simulink model "atrias_original"  (R2017a)
settings: Solver=ode45  StartTime=0.0  StopTime=sim_t  RelTol=1e-6  EnableMultiTasking=on
values from neighbouring files (symbols this model uses):
  N = grid_slice*1000    [createGrid.m]
  nm = fn_set_vnmc_params(sm, sample_time)    [kernel_scores_NM_mismatch.m]    (also in main_ATRIAS_cluster.m)
  nmc_BLCtrlPar = nmc.BLCtrlPar    [kernel_scores_NM_mismatch.m]    (also in main_ATRIAS_cluster.m)
  nmc_FPCtrlPar = nmc.FPCtrlPar    [kernel_scores_NM_mismatch.m]    (also in main_ATRIAS_cluster.m)
  nmc_LLCtrlPar = nmc.LLCtrlPar    [kernel_scores_NM_mismatch.m]    (also in main_ATRIAS_cluster.m)
  nmc_StCtrlPar = nmc.StCtrlPar    [kernel_scores_NM_mismatch.m]    (also in main_ATRIAS_cluster.m)
  nmc_SwCtrlPar = nmc.SwCtrlPar    [kernel_scores_NM_mismatch.m]    (also in main_ATRIAS_cluster.m)
  nmc_TrCtrlPar = nmc.TrCtrlPar    [kernel_scores_NM_mismatch.m]    (also in main_ATRIAS_cluster.m)
  nStep_switchCtrl = 10    [main_ATRIAS_cluster.m]
  nStep_thr = 1000    [createSimInitial.m]    (also in main_ATRIAS_cluster.m)
  rc_CtrlPar = [rc.k_placement, rc.T_step, rc.Cd, rc.kpt, rc.kdt, rc.desired_theta, rc.desired_z, rc.kpz, rc.kdz]    [kernel_scores_NM_mismatch.m]    (also in main_ATRIAS_cluster.m)
  sm = fn_set_MechParams(sm)    [kernel_scores_NM_mismatch.m]    (also in main_ATRIAS_cluster.m = fn_set_MechParams(sm,perturb))
  test_VNMC = 1    [createSimInitial.m]    (also in main_ATRIAS_cluster.m = 0)
undefined symbols (not defined in the file or in its folder): delta_phi_max, delta_phi_max_buffer, delta_phi_min, DiscIntNeverNeededParam, Discrete, idc, initial_dx_estimate, initial_dy_estimate, initial_dz_estimate, initial_z_estimate, kd_shin_max, kd_shin_min, kd_splay_max, kd_splay_min, kd_thigh_max, kd_thigh_min, kp_shin_max, kp_shin_min, kp_splay_max, kp_splay_min, kp_thigh_max, kp_thigh_min, mc, min_splay_angle, min_splay_buffer, phi_shin_max, phi_shin_max_buffer, phi_shin_min, phi_shin_min_buffer, phi_thigh_max, phi_thigh_max_buffer, phi_thigh_min, phi_thigh_min_buffer, rad, rc, s, sample_time, sgn, sim_d, t_friction, Time, X, Y, Z
libraries: sm_lib x202, nesl_utility x122, simulink x77, simulink_extras x24, fl_lib x16, mblibv1 x4, ctrlSharedLib x4, commnoisgen2 x1, dspswit3 x1
(part 7 of 17)

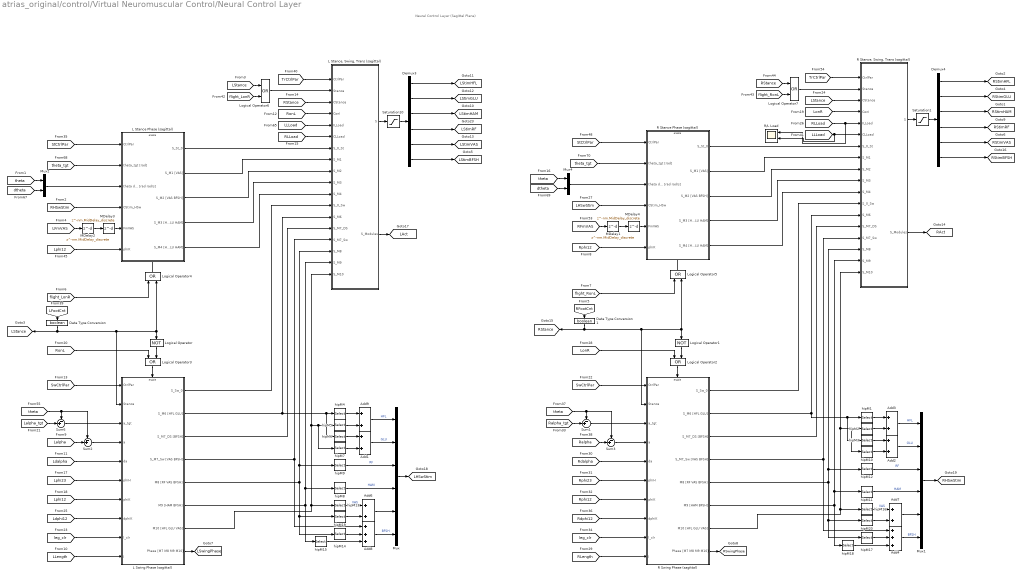
== system atrias_original/control/Virtual Neuromuscular Control/Neural Control Layer ==
  note: Neural Control Layer
      | (Sagittal Plane)
  Add{1..3,6..7,9} (6 alike) : Sum  Inputs=2
  Add4 : Sum  Inputs=3
  Add8 : Sum  Inputs=3
  Data Type Conversion : DataTypeConversion  OutDataTypeStr=boolean
  Data Type Conversion1 : DataTypeConversion  OutDataTypeStr=boolean
  Demux3 : Demux  Outputs=6
  Demux4 : Demux  Outputs=6
  L Stance Phase (sagittal) : Subsystem  TreatAsAtomicUnit=on
  "L Stance, Swing, Trans (sagittal)" : Subsystem
  L Swing Phase (sagittal) : Subsystem  TreatAsAtomicUnit=on
  Logical Operator : Logic  Operator=NOT  AllPortsSameDT=off  OutDataTypeStr=boolean
  Logical Operator1 : Logic  Operator=NOT  AllPortsSameDT=off  OutDataTypeStr=boolean
  Logical Operator{2..7} (6 alike) : Logic  Operator=OR  AllPortsSameDT=off  OutDataTypeStr=boolean
  MDelay{1..4} (4 alike) : Delay  DelayLength=nm.MidDelay_discrete  InitialCondition=0  SampleTime=sample_time
  Mux : Mux  Inputs=6
  Mux1 : Mux  Inputs=6
  Mux2 : Mux  Inputs=2
  Mux4 : Mux  Inputs=2
  R Stance Phase (sagittal) : Subsystem  TreatAsAtomicUnit=on
  "R Stance, Swing, Trans (sagittal)" : Subsystem
  R Swing Phase (sagittal) : Subsystem  TreatAsAtomicUnit=on
  R/L Load : Scope  NumInputPorts=2
  Saturation1 : Saturate  UpperLimit=1  LowerLimit=0.01  ZeroCross=off
  Saturation10 : Saturate  UpperLimit=1  LowerLimit=0.01  ZeroCross=off
  Sum{1..3,6} (4 alike) : Sum  Inputs=-+|
  hipM{1,4,8,11} (4 alike) : Selector  InputPortWidth=2  IndexOptions=Index vector (dialog)  Indices=1  OutputSizes=1
  hipM{7,10,19..20} (4 alike) : Selector  InputPortWidth=3  IndexOptions=Index vector (dialog)  Indices=2  OutputSizes=1
  hipM{2,5,9,12} (4 alike) : Selector  InputPortWidth=3  IndexOptions=Index vector (dialog)  Indices=1  OutputSizes=1
  hipM{13..14,16..17} (4 alike) : Selector  InputPortWidth=3  IndexOptions=Index vector (dialog)  Indices=3  OutputSizes=1
  hipM{3,6,15,18} (4 alike) : Selector  InputPortWidth=2  IndexOptions=Index vector (dialog)  Indices=2  OutputSizes=1
  tag scope: LAct=global, LHSwStim=global, LStance=global, LStimBFSH=global, LStimGLU=global, LStimHAM=global, LStimHFL=global, LStimRF=global, LStimVAS=global, LSwingPhase=global, RAct=global, RHSwStim=global, RStance=global, RStimBFSH=global, RStimGLU=global, RStimHAM=global, RStimHFL=global, RStimRF=global, RStimVAS=global, RSwingPhase=global
  wires:
  MDelay4/1 -> R Stance Phase (sagittal)/5(FmVAS)
  MDelay3/1 -> L Stance Phase (sagittal)/5(FmVAS)
  [RStance] -> "L Stance, Swing, Trans (sagittal)"/3(CStance)
  [RFootCnt] -> Data Type Conversion1/1
  [LFootCnt] -> Data Type Conversion/1
  [Rphi12] -> R Swing Phase (sagittal)/7(phiK)
  [Rphi23] -> R Swing Phase (sagittal)/6(phiH)
  [Rdphi12] -> R Swing Phase (sagittal)/8(dphiK)
  [Rdalpha] -> R Swing Phase (sagittal)/5(da)
  [RLength] -> R Swing Phase (sagittal)/10(l)
  Sum1/1 -> R Swing Phase (sagittal)/3(a_tgt)
  [theta] -> Sum3/1, Sum1/1
  [Ralpha_tgt] -> Sum1/2
  [leg_clr] -> R Swing Phase (sagittal)/9(l_clr)
  [Lphi12] -> L Swing Phase (sagittal)/7(phiK)
  [Lphi23] -> L Swing Phase (sagittal)/6(phiH)
  [Ldphi12] -> L Swing Phase (sagittal)/8(dphiK)
  [Ldalpha] -> L Swing Phase (sagittal)/5(da)
  [LLength] -> L Swing Phase (sagittal)/10(l)
  Add4/1 -> Mux1/6  "BFSH"
  hipM18/1 -> Add4/3
  hipM17/1 -> Add4/2
  R Swing Phase (sagittal)/3(S_M7_DS [BFSH]) -> "R Stance, Swing, Trans (sagittal)"/14(S_M7_DS)
  R Swing Phase (sagittal)/7(M10 [HFL GLU VAS]) -> "R Stance, Swing, Trans (sagittal)"/18(S_M10), hipM10/1, hipM2/1, hipM16/1
  R Swing Phase (sagittal)/5(M8 [RF VAS BFSH]) -> hipM20/1, hipM17/1, "R Stance, Swing, Trans (sagittal)"/16(S_M8), hipM12/1
  hipM15/1 -> Add8/3
  hipM14/1 -> Add8/2
  L Swing Phase (sagittal)/3(S_M7_DS [BFSH]) -> "L Stance, Swing, Trans (sagittal)"/14(S_M7_DS)
  Add8/1 -> Mux/6  "BFSH"
  "L Stance, Swing, Trans (sagittal)"/2(S_Modules) -> [LAct]
  "R Stance, Swing, Trans (sagittal)"/2(S_Modules) -> [RAct]
  R Swing Phase (sagittal)/8(Phase [M7 M8 M9 M10]) -> [RSwingPhase]
  L Swing Phase (sagittal)/8(Phase [M7 M8 M9 M10]) -> [LSwingPhase]
  hipM11/1 -> Mux1/4  "HAM"
  hipM12/1 -> Mux1/3  "RF"
  Add2/1 -> Mux1/2  "GLU"
  hipM10/1 -> Add2/2
  hipM3/1 -> Add2/1
  Add3/1 -> Mux1/1  "HFL"
  hipM2/1 -> Add3/2
  hipM1/1 -> Add3/1
  Mux1/1 -> [RHSwStim]
  R Swing Phase (sagittal)/6(M9 [HAM BFSH]) -> hipM18/1, "R Stance, Swing, Trans (sagittal)"/17(S_M9), hipM11/1
  R Swing Phase (sagittal)/2(S_M6 [HFL GLU]) -> hipM1/1, hipM3/1, "R Stance, Swing, Trans (sagittal)"/13(S_M6)
  R Swing Phase (sagittal)/1(S_Sw_0) -> "R Stance, Swing, Trans (sagittal)"/12(S_0_Sw)
  "R Stance, Swing, Trans (sagittal)"/1(S) -> Saturation1/1
  hipM8/1 -> Mux/4  "HAM"
  hipM9/1 -> Mux/3  "RF"
  Add1/1 -> Mux/2  "GLU"
  hipM7/1 -> Add1/2
  hipM6/1 -> Add1/1
  Add9/1 -> Mux/1  "HFL"
  hipM5/1 -> Add9/2
  hipM4/1 -> Add9/1
  Mux/1 -> [LHSwStim]
  L Swing Phase (sagittal)/7(M10 [HFL GLU VAS]) -> hipM7/1, hipM5/1, "L Stance, Swing, Trans (sagittal)"/18(S_M10), hipM13/1
  L Swing Phase (sagittal)/6(M9 [HAM BFSH]) -> hipM8/1, "L Stance, Swing, Trans (sagittal)"/17(S_M9), hipM15/1
  L Swing Phase (sagittal)/5(M8 [RF VAS BFSH]) -> hipM19/1, hipM14/1, hipM9/1, "L Stance, Swing, Trans (sagittal)"/16(S_M8)
  L Swing Phase (sagittal)/2(S_M6 [HFL GLU]) -> "L Stance, Swing, Trans (sagittal)"/13(S_M6), hipM4/1, hipM6/1
  L Stance Phase (sagittal)/5(S_M4 [HFL GLU HAM]) -> "L Stance, Swing, Trans (sagittal)"/11(S_M4)
  R Stance Phase (sagittal)/5(S_M4 [HFL GLU HAM]) -> "R Stance, Swing, Trans (sagittal)"/11(S_M4)
  Mux4/1 -> R Stance Phase (sagittal)/3(theta dtheta [rad rad/s])
  Mux2/1 -> L Stance Phase (sagittal)/3(theta dtheta [rad rad/s])
  [RLLoad] -> R/L Load/1, "R Stance, Swing, Trans (sagittal)"/5(ILLoad)
  R Stance Phase (sagittal)/4(S_M3 [HFL GLU HAM]) -> "R Stance, Swing, Trans (sagittal)"/10(S_M3)
  L Stance Phase (sagittal)/4(S_M3 [HFL GLU HAM]) -> "L Stance, Swing, Trans (sagittal)"/10(S_M3)
  [theta_tgt] -> R Stance Phase (sagittal)/2(theta_tgt [rad])
  [dtheta] -> Mux4/2
  [theta] -> Mux4/1
  [LLLoad] -> "L Stance, Swing, Trans (sagittal)"/5(ILLoad)
  [theta_tgt] -> L Stance Phase (sagittal)/2(theta_tgt [rad])
  [dtheta] -> Mux2/2
  [theta] -> Mux2/1
  R Stance Phase (sagittal)/3(S_M2 [VAS BFSH]) -> "R Stance, Swing, Trans (sagittal)"/9(S_M2)
  R Stance Phase (sagittal)/2(S_M1 [VAS]) -> "R Stance, Swing, Trans (sagittal)"/8(S_M1)
  L Stance Phase (sagittal)/3(S_M2 [VAS BFSH]) -> "L Stance, Swing, Trans (sagittal)"/9(S_M2)
  L Stance Phase (sagittal)/2(S_M1 [VAS]) -> "L Stance, Swing, Trans (sagittal)"/8(S_M1)
  R Stance Phase (sagittal)/1(S_St_0) -> "R Stance, Swing, Trans (sagittal)"/7(S_0_St)
  L Swing Phase (sagittal)/1(S_Sw_0) -> "L Stance, Swing, Trans (sagittal)"/12(S_0_Sw)
  L Stance Phase (sagittal)/1(S_St_0) -> "L Stance, Swing, Trans (sagittal)"/7(S_0_St)
  Sum6/1 -> L Swing Phase (sagittal)/3(a_tgt)
  [LStance] -> "R Stance, Swing, Trans (sagittal)"/3(CStance)
  Logical Operator7/1 -> "R Stance, Swing, Trans (sagittal)"/2(Stance)
  [theta] -> Sum2/1, Sum6/1
  [Lalpha_tgt] -> Sum6/2
  Demux4/6 -> [RStimBFSH]
  Demux4/5 -> [RStimVAS]
  Demux4/4 -> [RStimRF]
  Demux4/3 -> [RStimHAM]
  Demux4/2 -> [RStimGLU]
  Demux4/1 -> [RStimHFL]
  Demux3/6 -> [LStimBFSH]
  Demux3/5 -> [LStimVAS]
  Demux3/4 -> [LStimRF]
  Demux3/3 -> [LStimHAM]
  Demux3/2 -> [LStimGLU]
  Demux3/1 -> [LStimHFL]
  [RLLoad] -> "L Stance, Swing, Trans (sagittal)"/6(CLLoad)
  [LonR] -> "R Stance, Swing, Trans (sagittal)"/4(ConI)
  Saturation1/1 -> Demux4/1
  [LLLoad] -> R/L Load/2, "R Stance, Swing, Trans (sagittal)"/6(CLLoad)
  [TrCtrlPar] -> "R Stance, Swing, Trans (sagittal)"/1(CtrlPar)
  Logical Operator2/1 -> R Swing Phase (sagittal)/Enable
  Data Type Conversion1/1 -> [RStance], R Swing Phase (sagittal)/2(Stance), Logical Operator5/2, Logical Operator1/1
  [SwCtrlPar] -> R Swing Phase (sagittal)/1(CtrlPar)
  MDelay1/1 -> MDelay4/1
  [RFmVAS] -> MDelay1/1
  [LHSwStim] -> R Stance Phase (sagittal)/4(CStim_HSw)
  [StCtrlPar] -> R Stance Phase (sagittal)/1(CtrlPar)
  [RonL] -> "L Stance, Swing, Trans (sagittal)"/4(ConI)
  "L Stance, Swing, Trans (sagittal)"/1(S) -> Saturation10/1
  Saturation10/1 -> Demux3/1
  [TrCtrlPar] -> "L Stance, Swing, Trans (sagittal)"/1(CtrlPar)
  [leg_clr] -> L Swing Phase (sagittal)/9(l_clr)
  Logical Operator3/1 -> L Swing Phase (sagittal)/Enable
  Data Type Conversion/1 -> [LStance], L Swing Phase (sagittal)/2(Stance), Logical Operator/1, Logical Operator4/2
  [SwCtrlPar] -> L Swing Phase (sagittal)/1(CtrlPar)
  MDelay2/1 -> MDelay3/1
  [LFmVAS] -> MDelay2/1
  [RHSwStim] -> L Stance Phase (sagittal)/4(CStim_HSw)
  [StCtrlPar] -> L Stance Phase (sagittal)/1(CtrlPar)
  Add6/1 -> Mux/5
  hipM13/1 -> Add6/1  "VAS"
  hipM19/1 -> Add6/2
  L Swing Phase (sagittal)/4(S_M7_Sw [VAS BFSH]) -> "L Stance, Swing, Trans (sagittal)"/15(S_M7_Sw), Add8/1
  hipM20/1 -> Add7/2
  hipM16/1 -> Add7/1  "VAS"
  Add7/1 -> Mux1/5
  R Swing Phase (sagittal)/4(S_M7_Sw [VAS BFSH]) -> Add4/1, "R Stance, Swing, Trans (sagittal)"/15(S_M7_Sw)
  [Lalpha] -> Sum2/2
  Sum2/1 -> L Swing Phase (sagittal)/4(a)
  [Ralpha] -> Sum3/2
  Sum3/1 -> R Swing Phase (sagittal)/4(a)
  Logical Operator/1 -> Logical Operator3/2
  [RonL] -> Logical Operator3/1
  Logical Operator1/1 -> Logical Operator2/2
  [LonR] -> Logical Operator2/1
  Logical Operator5/1 -> R Stance Phase (sagittal)/Enable
  Logical Operator4/1 -> L Stance Phase (sagittal)/Enable
  [flight_LonR] -> Logical Operator4/1
  [flight_RonL] -> Logical Operator5/1
  [LStance] -> Logical Operator6/1
  Logical Operator6/1 -> "L Stance, Swing, Trans (sagittal)"/2(Stance)
  [flight_LonR] -> Logical Operator6/2
  [flight_RonL] -> Logical Operator7/2
  [RStance] -> Logical Operator7/1
  [Lphi12] -> L Stance Phase (sagittal)/6(phiK)
  [Rphi12] -> R Stance Phase (sagittal)/6(phiK)

== system atrias_original/control/Virtual Neuromuscular Control/Torque Distribution ==
  note: J^(-T) [tauB; tauF] = [tauH, tauK]
  note: Map Torques
  note: J^(-T) [tauB; tauF] = [tauH, tauK]
  R tauK_des [Nm] : Inport
  R tauH_des [Nm] : Inport  Port=2
  R Jacobian Constant (k) : Inport  Port=3
  L tauK_des [Nm] : Inport  Port=4
  L tauH_des [Nm] : Inport  Port=5
  L Jacobian Constant (k) : Inport  Port=6
  Demux : Demux
  Demux1 : Demux  Outputs=2
  Demux2 : Demux  Outputs=2
  L H/K torques : Scope  NumInputPorts=2
  Mux : Mux
  Mux1 : Mux  Inputs=2
  Mux2 : Mux  Inputs=2
  "R H/K torques " : Scope  NumInputPorts=2
  Switch1 : Switch  Criteria=u2 > Threshold
  Switch2 : Switch  Criteria=u2 > Threshold
  Torque Limiter (outside) {1,3..5} (4 alike) : Saturate  UpperLimit=mc.LEG_MTR_MAX_TORQUE  LowerLimit=-mc.LEG_MTR_MAX_TORQUE
      settings: AttributesFormatString=Hi: %<UpperLimit>\nLo: %<LowerLimit>
  map_tau_L : MATLAB Function  TreatAsAtomicUnit=on
  map_tau_R : MATLAB Function  TreatAsAtomicUnit=on
  mech limit avoidance1 : Subsystem  Commented=on
  R tauB [Nm] : Outport
  R tauF [Nm] : Outport  Port=2
  R J_inv_transpose [2x2] : Outport  Port=3
  L tauB [Nm] : Outport  Port=4
  L tauF [Nm] : Outport  Port=5
  L J_inv_transpose [2x2] : Outport  Port=6
  wires:
  R Jacobian Constant (k)/1 -> map_tau_R/3(k)
  map_tau_R/3(Jinv_trans) -> R J_inv_transpose [2x2]/1
  L Jacobian Constant (k)/1 -> map_tau_L/3(k)
  map_tau_L/3(Jinv_trans) -> L J_inv_transpose [2x2]/1
  map_tau_L/1(tauB) -> Mux2/1
  map_tau_L/2(tauF) -> Mux2/2
  Mux/1 -> Demux/1
  Demux/1 -> [RtauH]
  R tauH_des [Nm]/1 -> Mux/1
  R tauK_des [Nm]/1 -> Mux/2
  L tauH_des [Nm]/1 -> Mux/3
  L tauK_des [Nm]/1 -> Mux/4
  Demux/2 -> [RtauK]
  Demux/3 -> [LtauH]
  Demux/4 -> [LtauK]
  [RtauH] -> "R H/K torques "/1, map_tau_R/1(tauH_des)
  [RtauK] -> "R H/K torques "/2, map_tau_R/2(tauK_des)
  [LtauH] -> L H/K torques/1, map_tau_L/1(tauH_des)
  Switch1/1 -> Demux1/1
  [LFootCnt] -> Switch1/2
  Mux2/1 -> Torque Limiter (outside) 3/1, Torque Limiter (outside) 1/1
  Torque Limiter (outside) 3/1 -> Switch1/3
  Torque Limiter (outside) 1/1 -> Switch1/1
  Demux1/2 -> L tauF [Nm]/1
  Demux1/1 -> L tauB [Nm]/1
  map_tau_R/1(tauB) -> Mux1/1
  map_tau_R/2(tauF) -> Mux1/2
  Switch2/1 -> Demux2/1
  [RFootCnt] -> Switch2/2
  Mux1/1 -> Torque Limiter (outside) 5/1, Torque Limiter (outside) 4/1
  Torque Limiter (outside) 4/1 -> Switch2/3
  Torque Limiter (outside) 5/1 -> Switch2/1
  Demux2/2 -> R tauF [Nm]/1
  Demux2/1 -> R tauB [Nm]/1
  [LtauK] -> L H/K torques/2, map_tau_L/2(tauK_des)

== system atrias_original/ATRIAS_sim/Mechanical System Layer/Boom/Frame Data ==
  Kinematic Data : ToWorkspace  VariableName=boom_roll_out  SampleTime=sm.output_sample_time
      settings: Save2DSignal=2-D array (concatenate along first dimension)
  Mux : Mux
  PS-Simulink Converter{,1..3} (4 alike) : nesl_utility/PS-Simulink Converter  PhysicalDomain=network_engine_domain  SubClassName=ps_output  LeftPortType=input  RightPortType=output  PseudoPeriodic=off  Frequencies=[]  Unit=1  AffineConversion=off
  Transform Sensor : sm_lib/Frames and Transforms/Transform Sensor  MeasurementFrame=World  SenseAngle=off  SenseAxis=off  SenseAngle1=off  SenseAngle2=off  SenseAngle3=off  SenseQ=on  SenseR=off  SenseOmegaX=off  SenseOmegaY=off  SenseOmegaZ=off  SenseOmega1=off  SenseOmega2=off  SenseOmega3=off  SenseQDot=off  SenseRDot=off  SenseAlphaX=off  SenseAlphaY=off  SenseAlphaZ=off  SenseAlpha1=off  SenseAlpha2=off  SenseAlpha3=off  SenseQDDot=off  SenseRDDot=off  SenseX=on  SenseY=on  SenseZ=on  SenseRad=off  SenseAzim=off  SenseDist=off  SenseInc=off  SenseXDot=off  SenseYDot=off  SenseZDot=off  SenseRadDot=off  SenseAzimDot=off  SenseDistDot=off  SenseIncDot=off  SenseXDDot=off  SenseYDDot=off  SenseZDDot=off  SenseRadDDot=off  SenseAzimDDot=off  SenseDistDDot=off  SenseIncDDot=off
  World Frame : sm_lib/Frames and Transforms/World Frame
  Frame : PMIOPort  Port=1  Side=Left
  wires:
  Mux/1 -> Kinematic Data/1
  PS-Simulink Converter/1 -> Mux/1
  PS-Simulink Converter1/1 -> Mux/2
  PS-Simulink Converter2/1 -> Mux/3
  PS-Simulink Converter3/1 -> Mux/4
  connections:
  PS-Simulink Converter3/LConn1 -- Transform Sensor/RConn5
  PS-Simulink Converter2/LConn1 -- Transform Sensor/RConn4
  PS-Simulink Converter1/LConn1 -- Transform Sensor/RConn3
  PS-Simulink Converter/LConn1 -- Transform Sensor/RConn2
  Transform Sensor/RConn1 -- Frame/RConn1
  Transform Sensor/LConn1 -- World Frame/RConn1

== system atrias_original/ATRIAS_sim/Mechanical System Layer/L Ground Contact/Angle Range Map1 ==
  "[-pi, pi]" : Inport
  Constant : Constant  Value=2*pi
  Sum3 : Sum  Inputs=|++
  Switch : Switch  ZeroCross=off
  "[0,2*pi]" : Outport
  wires:
  Switch/1 -> "[0,2*pi]"/1
  Constant/1 -> Sum3/2
  Sum3/1 -> Switch/3
  "[-pi, pi]"/1 -> Switch/2, Switch/1, Sum3/1

== system atrias_original/ATRIAS_sim/Mechanical System Layer/L Ground Contact/Ground Friction Model ==
  note: Normal Ground Stiction Model
  note: Transverse Ground Friction Model
  delta normal [m] : Inport
  vnormal [m/s] : Inport  Port=2
  x [m] : Inport  Port=3
  vx [m/s] : Inport  Port=4
  z [m] : Inport  Port=5
  vz [m/s] : Inport  Port=6
  Contact! : EnablePort  StatesWhenEnabling=reset
  Data Type Conversion : DataTypeConversion  OutDataTypeStr=double
  Friction Switch : Subsystem
  Gain3 : Gain  Gain=sm.k_gy
  Gain4 : Gain  Gain=1/sm.v_gy_max
  Logical Operator : Logic  Operator=NOT  AllPortsSameDT=off  OutDataTypeStr=boolean
  Mux1 : Mux  Inputs=2
  Sum1 : Sum
  Sum2 : Sum
  normal-Axis Ground Force : Fcn  Expr="- u(1)  *  (1-u(2)) * (u(2)<1)"
  t-Axis Kinetic Friction Model : Subsystem
  t-Axis Static Friction Model : Subsystem
  FxFriction [N] : Outport  OutputWhenDisabled=reset  InitialOutput=0
      settings: AttributesFormatString=initial = '%<InitialOutput>'\nwhen\ndisabled\n'%<OutputWhenDisabled>'
  FyFriction [N] : Outport  Port=2  OutputWhenDisabled=reset  InitialOutput=0
      settings: AttributesFormatString=initial = '%<InitialOutput>'\nwhen\ndisabled\n'%<OutputWhenDisabled>'
  Fn_Ground[N] : Outport  Port=3  OutputWhenDisabled=reset  InitialOutput=0
      settings: AttributesFormatString=initial = '%<InitialOutput>'\nwhen disabled = '%<OutputWhenDisabled>'
  Stiction! : Outport  Port=4  OutputWhenDisabled=reset  InitialOutput=0
      settings: AttributesFormatString=initial = '%<InitialOutput>'\nwhen\ndisabled\n'%<OutputWhenDisabled>'
  wires:
  Data Type Conversion/1 -> Stiction!/1
  vz [m/s]/1 -> t-Axis Static Friction Model/5(vel_z [m/s]), t-Axis Kinetic Friction Model/4(vel_z [m/s])
  z [m]/1 -> t-Axis Kinetic Friction Model/3(pos_z [m]), t-Axis Static Friction Model/4(pos_z [m])
  t-Axis Kinetic Friction Model/2(posFP_z [m]) -> t-Axis Static Friction Model/7(posFP_z [m])
  Sum2/1 -> FyFriction [N]/1
  t-Axis Kinetic Friction Model/5(Fz_Slide [N]) -> Sum2/2
  t-Axis Static Friction Model/1(Fz_Stick [N]) -> Sum2/1
  Gain4/1 -> Mux1/2
  Gain3/1 -> Mux1/1
  Mux1/1 -> normal-Axis Ground Force/1
  Logical Operator/1 -> t-Axis Kinetic Friction Model/Enable
  t-Axis Kinetic Friction Model/3(Stiction!) -> Friction Switch/2(Stick!)
  t-Axis Static Friction Model/3(Sliding!) -> Friction Switch/1(Slide!)
  Friction Switch/1(Stiction) -> t-Axis Static Friction Model/Enable, Logical Operator/1, Data Type Conversion/1
  Sum1/1 -> FxFriction [N]/1
  t-Axis Static Friction Model/2(Fx_Stick [N]) -> Sum1/1
  t-Axis Kinetic Friction Model/4(Fx_Slide [N]) -> Sum1/2
  t-Axis Kinetic Friction Model/1(posFP_x [m]) -> t-Axis Static Friction Model/6(posFP_x [m])
  vx [m/s]/1 -> t-Axis Static Friction Model/3(vel_x [m/s]), t-Axis Kinetic Friction Model/2(vel_x [m/s])
  x [m]/1 -> t-Axis Static Friction Model/2(pos_x [m]), t-Axis Kinetic Friction Model/1(pos_x [m])
  vnormal [m/s]/1 -> Gain4/1
  delta normal [m]/1 -> Gain3/1
  normal-Axis Ground Force/1 -> Fn_Ground[N]/1, t-Axis Kinetic Friction Model/5(F_Normal [N]), t-Axis Static Friction Model/1(F_Normal [N])

== system atrias_original/ATRIAS_sim/Mechanical System Layer/L Ground Contact/Tranverse Component ==
  "x, y, z" : Inport
  boom yaw [rad] : Inport  Port=2
  Demux1 : Demux  Outputs=3
  Product : Product
  Product1 : Product
  Sum2 : Sum  Inputs=+|+
  Terminator1 : Terminator
  Trigonometric Function1 : Trigonometry  Operator=cos
  Trigonometric Function2 : Trigonometry
  transverse : Outport
  wires:
  Trigonometric Function2/1 -> Product1/1
  Demux1/2 -> Product1/2
  Demux1/1 -> Product/1
  Sum2/1 -> transverse/1
  Product/1 -> Sum2/1
  boom yaw [rad]/1 -> Trigonometric Function1/1, Trigonometric Function2/1
  Trigonometric Function1/1 -> Product/2
  Product1/1 -> Sum2/2
  "x, y, z"/1 -> Demux1/1
  Demux1/3 -> Terminator1/1

== system atrias_original/ATRIAS_sim/Mechanical System Layer/L Hip Shaft/Frame Data ==
  Kinematic Data : ToWorkspace  VariableName=l_hip_out  SampleTime=sm.output_sample_time
      settings: Save2DSignal=2-D array (concatenate along first dimension)
  Mux : Mux
  PS-Simulink Converter{,1..3} (4 alike) : nesl_utility/PS-Simulink Converter  PhysicalDomain=network_engine_domain  SubClassName=ps_output  LeftPortType=input  RightPortType=output  PseudoPeriodic=off  Frequencies=[]  Unit=1  AffineConversion=off
  Transform Sensor : sm_lib/Frames and Transforms/Transform Sensor  MeasurementFrame=World  SenseAngle=off  SenseAxis=off  SenseAngle1=off  SenseAngle2=off  SenseAngle3=off  SenseQ=on  SenseR=off  SenseOmegaX=off  SenseOmegaY=off  SenseOmegaZ=off  SenseOmega1=off  SenseOmega2=off  SenseOmega3=off  SenseQDot=off  SenseRDot=off  SenseAlphaX=off  SenseAlphaY=off  SenseAlphaZ=off  SenseAlpha1=off  SenseAlpha2=off  SenseAlpha3=off  SenseQDDot=off  SenseRDDot=off  SenseX=on  SenseY=on  SenseZ=on  SenseRad=off  SenseAzim=off  SenseDist=off  SenseInc=off  SenseXDot=off  SenseYDot=off  SenseZDot=off  SenseRadDot=off  SenseAzimDot=off  SenseDistDot=off  SenseIncDot=off  SenseXDDot=off  SenseYDDot=off  SenseZDDot=off  SenseRadDDot=off  SenseAzimDDot=off  SenseDistDDot=off  SenseIncDDot=off
  World Frame : sm_lib/Frames and Transforms/World Frame
  Frame : PMIOPort  Port=1  Side=Left
  wires:
  Mux/1 -> Kinematic Data/1
  PS-Simulink Converter/1 -> Mux/1
  PS-Simulink Converter1/1 -> Mux/2
  PS-Simulink Converter2/1 -> Mux/3
  PS-Simulink Converter3/1 -> Mux/4
  connections:
  PS-Simulink Converter3/LConn1 -- Transform Sensor/RConn5
  PS-Simulink Converter2/LConn1 -- Transform Sensor/RConn4
  PS-Simulink Converter1/LConn1 -- Transform Sensor/RConn3
  PS-Simulink Converter/LConn1 -- Transform Sensor/RConn2
  Transform Sensor/RConn1 -- Frame/RConn1
  Transform Sensor/LConn1 -- World Frame/RConn1

== system atrias_original/ATRIAS_sim/Mechanical System Layer/L Leg/Angle Range Map ==
  "[-pi, pi]" : Inport
  Constant : Constant  Value=2*pi
  Sum3 : Sum  Inputs=|++
  Switch : Switch  ZeroCross=off
  "[0,2*pi]" : Outport
  wires:
  Switch/1 -> "[0,2*pi]"/1
  Constant/1 -> Sum3/2
  Sum3/1 -> Switch/3
  "[-pi, pi]"/1 -> Switch/2, Switch/1, Sum3/1

== system atrias_original/ATRIAS_sim/Mechanical System Layer/L Leg/Angle Range Map1 ==
  "[-pi, pi]" : Inport
  Constant : Constant  Value=2*pi
  Sum3 : Sum  Inputs=|++
  Switch : Switch  ZeroCross=off
  "[0,2*pi]" : Outport
  wires:
  "[-pi, pi]"/1 -> Sum3/1, Switch/1, Switch/2
  Sum3/1 -> Switch/3
  Constant/1 -> Sum3/2
  Switch/1 -> "[0,2*pi]"/1

== system atrias_original/ATRIAS_sim/Mechanical System Layer/L Leg/Four Bar Link ==
  CS1 to CS2 : sm_lib/Frames and Transforms/Rigid Transform  TranslationMethod=Cartesian  TranslationStandardOffset=0  TranslationLengthUnit=m  TranslationStandardAxis=+Z  TranslationCartesianOffset=[0 -sm.l_seg 0]  TranslationROffset=0  TranslationROffsetUnits=m  TranslationZOffset=0  TranslationZOffsetUnits=m  TranslationThetaOffset=0  TranslationThetaOffsetUnits=deg  RotationMethod=None  RotationAngleUnits=deg  RotationStandardAxis=+Z  RotationAngle=0  RotationArbitraryAxis=[0 0 1]  FollAlignAxisA=+X  BaseAlignAxisA=+Y  FollAlignAxisB=+Y  BaseAlignAxisB=+Z  RotationSequenceAxes=FollowerAxes  RotationSequence=XYX  RotationSequenceAngles=[0 0 0]  RotationSequenceAnglesUnits=deg  RotationMatrix=[1 0 0; 0 1 0; 0 0 1]
  Frame Data : Subsystem
  Solid : sm_lib/Body Elements/Solid  InertiaType=Custom  Mass=sm.m_fblink  MassUnits=kg  CenterOfMass=sm.com_fblink  CenterOfMassUnits=m  MomentsOfInertia=sm.i_fblink_moments  MomentsOfInertiaUnits=kg*m^2  ProductsOfInertia=sm.i_fblink_products  ProductsOfInertiaUnits=kg*m^2  DensityBased=on  Density=1000  DensityUnits=kg/(m^3)  DoExposeReferenceFrame=on  SerializedFrames=<Frames/>  GraphicType=FromGeometry  MarkerShape=Sphere  MarkerSize=10  MarkerSizeUnits=m  GraphicVisPropType=AdvancedVisualProperties  GraphicDiffuseColor=sm.fblink_color_d  GraphicSpecularColor=[0.5 0.5 0.5 1.0]  GraphicAmbientColor=[sm.fblink_color_d*0.5 1.0]  GraphicEmissiveColor=[0.0 0.0 0.0 1.0]  GraphicShininess=128  GraphicOpacity=1.0  GeometryShape=FromFile  RectangleSize=[1 1]  RectangleSizeUnits=m  BrickDimensions="[0.1  1 0.1]"  BrickDimensionUnits=m  CylinderRadius=1  CylinderRadiusUnits=m  CylinderLength=1  CylinderLengthUnits=m  SphereRadius=1  SphereRadiusUnits=m  EllipsoidRadii=[1 1 1]  EllipsoidRadiiUnits=m  ExtrusionCrossSection=[1 1; -1 1; -1 -1; 1 -1]  ExtrusionCrossSectionUnits=m  ExtrusionLength=1  ExtrusionLengthUnits=m  PolygonNumSides=3  PolygonOuterRadius=1  PolygonOuterRadiusUnits=m  ExtGeomFileType=STL  ExtGeomFileName=../models/four_bar_link.stl  ExtGeomFileUnits=m  RevolutionCrossSection=[1 1; 1 -1; 2 -1; 2 1]  RevolutionCrossSectionUnits=m  RevolutionExtent=Full  RevolutionAngle=180  RevolutionAngleUnits=deg
  CS1 : PMIOPort  Port=1  Side=Left
  CS2 : PMIOPort  Port=2  Side=Right
  connections:
  CS1 to CS2/LConn1 -- Frame Data/LConn1 -- CS1/RConn1 -- Solid/RConn1
  CS2/RConn1 -- CS1 to CS2/RConn1

== system atrias_original/ATRIAS_sim/Mechanical System Layer/L Leg/Lower Leg ==
  CS1 to CS2 : sm_lib/Frames and Transforms/Rigid Transform  TranslationMethod=Cartesian  TranslationStandardOffset=0  TranslationLengthUnit=m  TranslationStandardAxis=+Z  TranslationCartesianOffset=[0 -sm.lowerleg_12 0]  TranslationROffset=0  TranslationROffsetUnits=m  TranslationZOffset=0  TranslationZOffsetUnits=m  TranslationThetaOffset=0  TranslationThetaOffsetUnits=deg  RotationMethod=None  RotationAngleUnits=deg  RotationStandardAxis=+Z  RotationAngle=0  RotationArbitraryAxis=[0 0 1]  FollAlignAxisA=+X  BaseAlignAxisA=+Y  FollAlignAxisB=+Y  BaseAlignAxisB=+Z  RotationSequenceAxes=FollowerAxes  RotationSequence=XYX  RotationSequenceAngles=[0 0 0]  RotationSequenceAnglesUnits=deg  RotationMatrix=[1 0 0; 0 1 0; 0 0 1]
  CS1 to CS3 : sm_lib/Frames and Transforms/Rigid Transform  TranslationMethod=Cartesian  TranslationStandardOffset=0  TranslationLengthUnit=m  TranslationStandardAxis=+Z  TranslationCartesianOffset=[0 -sm.l_seg 0]  TranslationROffset=0  TranslationROffsetUnits=m  TranslationZOffset=0  TranslationZOffsetUnits=m  TranslationThetaOffset=0  TranslationThetaOffsetUnits=deg  RotationMethod=None  RotationAngleUnits=deg  RotationStandardAxis=+Z  RotationAngle=0  RotationArbitraryAxis=[0 0 1]  FollAlignAxisA=+X  BaseAlignAxisA=+Y  FollAlignAxisB=+Y  BaseAlignAxisB=+Z  RotationSequenceAxes=FollowerAxes  RotationSequence=XYX  RotationSequenceAngles=[0 0 0]  RotationSequenceAnglesUnits=deg  RotationMatrix=[1 0 0; 0 1 0; 0 0 1]
  Frame Data : Subsystem
  Solid : sm_lib/Body Elements/Solid  InertiaType=Custom  Mass=sm.m_lowerleg  MassUnits=kg  CenterOfMass=sm.com_lowerleg  CenterOfMassUnits=m  MomentsOfInertia=sm.i_lowerleg_moments  MomentsOfInertiaUnits=kg*m^2  ProductsOfInertia=sm.i_lowerleg_products  ProductsOfInertiaUnits=kg*m^2  DensityBased=on  Density=1000  DensityUnits=kg/(m^3)  DoExposeReferenceFrame=on  SerializedFrames=<Frames/>  GraphicType=FromGeometry  MarkerShape=Sphere  MarkerSize=10  MarkerSizeUnits=m  GraphicVisPropType=AdvancedVisualProperties  GraphicDiffuseColor=sm.lowerleg_color_d  GraphicSpecularColor=[0.5 0.5 0.5 1.0]  GraphicAmbientColor=[sm.lowerleg_color_d*0.5 1.0]  GraphicEmissiveColor=[0.0 0.0 0.0 1.0]  GraphicShininess=128  GraphicOpacity=1.0  GeometryShape=FromFile  RectangleSize=[1 1]  RectangleSizeUnits=m  BrickDimensions=[0.1 1 0.1]  BrickDimensionUnits=m  CylinderRadius=1  CylinderRadiusUnits=m  CylinderLength=1  CylinderLengthUnits=m  SphereRadius=1  SphereRadiusUnits=m  EllipsoidRadii=[1 1 1]  EllipsoidRadiiUnits=m  ExtrusionCrossSection=[1 1; -1 1; -1 -1; 1 -1]  ExtrusionCrossSectionUnits=m  ExtrusionLength=1  ExtrusionLengthUnits=m  PolygonNumSides=3  PolygonOuterRadius=1  PolygonOuterRadiusUnits=m  ExtGeomFileType=STL  ExtGeomFileName=../models/lower_leg.stl  ExtGeomFileUnits=m  RevolutionCrossSection=[1 1; 1 -1; 2 -1; 2 1]  RevolutionCrossSectionUnits=m  RevolutionExtent=Full  RevolutionAngle=180  RevolutionAngleUnits=deg
  CS1 : PMIOPort  Port=1  Side=Left
  CS2 : PMIOPort  Port=2  Side=Right
  CS3 : PMIOPort  Port=3  Side=Right
  connections:
  CS2/RConn1 -- CS1 to CS2/RConn1
  CS1/RConn1 -- Frame Data/LConn1 -- Solid/RConn1 -- CS1 to CS2/LConn1 -- CS1 to CS3/LConn1
  CS3/RConn1 -- CS1 to CS3/RConn1

== system atrias_original/ATRIAS_sim/Mechanical System Layer/L Leg/Mechanical Limits ==
  note: Mechanical Limits Model
  note: Thigh-Shin Collision
  note: Thigh-Shin Flexion Collision
  dphi_shin : Inport
  phi_shin : Inport  Port=2
  dphi_thigh : Inport  Port=3
  phi_thigh : Inport  Port=4
  Compare To Constant5 : simulink/Logic and Bit Operations/Compare To Constant  relop=<=  const=sm.phi_max_collision  OutDataTypeStr=boolean  ZeroCross=off
  Compare To Zero{,1..5} (6 alike) : simulink/Logic and Bit Operations/Compare To Zero  relop=<=  OutDataTypeStr=boolean  ZeroCross=off
  Constant : Constant  Value=sm.delta_phi_min
  Constant1 : Constant  Value=sm.phi_shin_max
  Constant2 : Constant  Value=sm.phi_thigh_min
  Constant3 : Constant  Value=sm.delta_phi_max
  Constant4 : Constant  Value=sm.phi_shin_min
  Constant5 : Constant  Value=sm.phi_thigh_max
  Enabled Subsystem : Subsystem  TreatAsAtomicUnit=on
  Gain : Gain  Gain=-1
  Gain1 : Gain  Gain=-1
  Gain2 : Gain  Gain=-1
  Logical Operator : Logic  Operator=OR  Inputs=1  AllPortsSameDT=off  OutDataTypeStr=boolean
  Mux : Mux  Inputs=6
  Shin Max Collision Model : Subsystem
  Shin Min Collision Model : Subsystem
  Stop Simulation6 : Stop
  Sum{1..3,5,7} (5 alike) : Sum  Inputs=-+|
  Sum10 : Sum  Inputs=+-|
  Sum11 : Sum  Inputs=-|+
  Sum4 : Sum  Inputs=+-|
  Sum6 : Sum  Inputs=+|-
  Sum8 : Sum  Inputs=+-|
  Sum9 : Sum  Inputs=-|+
  Thigh Max Collision Model : Subsystem
  Thigh Min Collision Model : Subsystem
  Thigh-Shin Collision Model : Subsystem
  Thigh-Shin Collision Model1 : Subsystem
  tau_shin_col : Outport
  tau_thigh_shin_col : Outport  Port=2
  tau_thigh_col : Outport  Port=3
  wires:
  Compare To Zero/1 -> Thigh-Shin Collision Model/Enable
  Sum1/1 -> Sum8/2, Sum3/2
  phi_shin/1 -> Sum1/2, Sum7/2, Sum4/2
  Sum2/1 -> Gain2/1, Thigh-Shin Collision Model/2(vphi [rad/s])
  Constant/1 -> Sum3/1
  Sum3/1 -> [col_r_leg_extension], Compare To Zero/1, Thigh-Shin Collision Model/1(delta_phi [rad])
  Compare To Zero1/1 -> Shin Max Collision Model/Enable
  Constant1/1 -> Sum4/1
  phi_thigh/1 -> Sum10/2, Sum5/2, Sum1/1
  dphi_thigh/1 -> Thigh Min Collision Model/2(vphi [rad/s]), Gain1/1, Sum2/1
  Constant2/1 -> Sum5/1
  Sum5/1 -> [col_thigh_min], Compare To Zero2/1, Thigh Min Collision Model/1(phi [rad])
  Gain/1 -> Shin Max Collision Model/2(vphi [rad/s])
  Compare To Zero2/1 -> Thigh Min Collision Model/Enable
  Compare To Zero3/1 -> Thigh-Shin Collision Model1/Enable
  Constant3/1 -> Sum8/1
  Sum8/1 -> [col_r_leg_flexion], Compare To Zero3/1, Thigh-Shin Collision Model1/1(delta_phi [rad])
  Thigh-Shin Collision Model/1(tau_interaction[Nm]) -> Sum6/1
  Thigh-Shin Collision Model1/1(tau_interaction[Nm]) -> Sum6/2
  Gain2/1 -> Thigh-Shin Collision Model1/2(vphi [rad/s])
  Compare To Zero4/1 -> Shin Min Collision Model/Enable
  Constant4/1 -> Sum7/1
  Sum7/1 -> [col_shin_min], Compare To Zero4/1, Shin Min Collision Model/1(phi [rad])
  dphi_shin/1 -> Sum2/2, Gain/1, Shin Min Collision Model/2(vphi [rad/s])
  Sum9/1 -> tau_shin_col/1
  Shin Max Collision Model/1(tau_interaction[Nm]) -> Sum9/1
  Shin Min Collision Model/1(tau_interaction[Nm]) -> Sum9/2
  Sum6/1 -> tau_thigh_shin_col/1
  Constant5/1 -> Sum10/1
  Compare To Zero5/1 -> Thigh Max Collision Model/Enable
  Sum11/1 -> tau_thigh_col/1
  Thigh Min Collision Model/1(tau_interaction[Nm]) -> Sum11/2
  Gain1/1 -> Thigh Max Collision Model/2(vphi [rad/s])
  Thigh Max Collision Model/1(tau_interaction[Nm]) -> Sum11/1
  [col_thigh_max] -> Mux/1
  [col_thigh_min] -> Mux/2
  [col_shin_max] -> Mux/3
  [col_shin_min] -> Mux/4
  [col_leg_extension] -> Mux/5
  [col_r_leg_flexion] -> Mux/6
  Mux/1 -> Compare To Constant5/1
  Logical Operator/1 -> Stop Simulation6/1, Enabled Subsystem/Enable
  Sum10/1 -> Thigh Max Collision Model/1(phi [rad]), Compare To Zero5/1, [col_thigh_max]
  Sum4/1 -> [col_shin_max], Compare To Zero1/1, Shin Max Collision Model/1(phi [rad])
  Compare To Constant5/1 -> Enabled Subsystem/1(Col_Flags), Logical Operator/1

== system atrias_original/ATRIAS_sim/Mechanical System Layer/L Leg/Shin ==
  CS1 to CS2 : sm_lib/Frames and Transforms/Rigid Transform  TranslationMethod=Cartesian  TranslationStandardOffset=0  TranslationLengthUnit=m  TranslationStandardAxis=+Z  TranslationCartesianOffset=[0 -sm.shin_12 0]  TranslationROffset=0  TranslationROffsetUnits=m  TranslationZOffset=0  TranslationZOffsetUnits=m  TranslationThetaOffset=0  TranslationThetaOffsetUnits=deg  RotationMethod=None  RotationAngleUnits=deg  RotationStandardAxis=+Z  RotationAngle=0  RotationArbitraryAxis=[0 0 1]  FollAlignAxisA=+X  BaseAlignAxisA=+Y  FollAlignAxisB=+Y  BaseAlignAxisB=+Z  RotationSequenceAxes=FollowerAxes  RotationSequence=XYX  RotationSequenceAngles=[0 0 0]  RotationSequenceAnglesUnits=deg  RotationMatrix=[1 0 0; 0 1 0; 0 0 1]
  Frame Data : Subsystem
  Solid : sm_lib/Body Elements/Solid  InertiaType=Custom  Mass=sm.m_shin  MassUnits=kg  CenterOfMass=sm.com_shin  CenterOfMassUnits=m  MomentsOfInertia=sm.i_shin_moments  MomentsOfInertiaUnits=kg*m^2  ProductsOfInertia=sm.i_shin_products  ProductsOfInertiaUnits=kg*m^2  DensityBased=on  Density=1000  DensityUnits=kg/(m^3)  DoExposeReferenceFrame=on  SerializedFrames=<Frames/>  GraphicType=FromGeometry  MarkerShape=Sphere  MarkerSize=10  MarkerSizeUnits=m  GraphicVisPropType=AdvancedVisualProperties  GraphicDiffuseColor=sm.shin_color_d  GraphicSpecularColor=[0.5 0.5 0.5 1.0]  GraphicAmbientColor=[sm.shin_color_d*0.5 1.0]  GraphicEmissiveColor=[0.0 0.0 0.0 1.0]  GraphicShininess=128  GraphicOpacity=1.0  GeometryShape=FromFile  RectangleSize=[1 1]  RectangleSizeUnits=m  BrickDimensions=[1 1 1]  BrickDimensionUnits=m  CylinderRadius=1  CylinderRadiusUnits=m  CylinderLength=1  CylinderLengthUnits=m  SphereRadius=1  SphereRadiusUnits=m  EllipsoidRadii=[1 1 1]  EllipsoidRadiiUnits=m  ExtrusionCrossSection=[1 1; -1 1; -1 -1; 1 -1]  ExtrusionCrossSectionUnits=m  ExtrusionLength=1  ExtrusionLengthUnits=m  PolygonNumSides=3  PolygonOuterRadius=1  PolygonOuterRadiusUnits=m  ExtGeomFileType=STL  ExtGeomFileName=../models/shin.stl  ExtGeomFileUnits=m  RevolutionCrossSection=[1 1; 1 -1; 2 -1; 2 1]  RevolutionCrossSectionUnits=m  RevolutionExtent=Full  RevolutionAngle=180  RevolutionAngleUnits=deg
  CS1 : PMIOPort  Port=1  Side=Left
  CS2 : PMIOPort  Port=2  Side=Right
  connections:
  CS2/RConn1 -- CS1 to CS2/RConn1
  Solid/RConn1 -- Frame Data/LConn1 -- CS1/RConn1 -- CS1 to CS2/LConn1

== system atrias_original/ATRIAS_sim/Mechanical System Layer/L Leg/Shin SEA ==
  note: Shin SEA Mechanics
  Shin Gear Torque [Nm] : Inport
  Shin Joint [rad rad/s] : Inport  Port=2
  Continuous Angle : mblibv1/Utilities/Continuous Angle  rad=rad  rads=rad/s
      settings: SourceProductName=Simscape Multibody  SourceProductBaseCode=MS
  Demux : Demux  Outputs=2
  Gain : Gain  Gain=sm.k_leg_spring
  Gain1 : Gain  Gain=sm.b_leg_spring
  Initial Gear Angle : Constant  Value=sm.shin_initial_l-sm.initial_deflection_l
  Inverse Gear Ratio1 : Gain  Gain=1/sm.N
  Inverse Gear Ratio2 : Gain  Gain=sm.Kt_leg
  Inverse Gear Ratio3 : Gain  Gain=1/sm.Kt_leg
  Motor Direction : Gain  Gain=-1
  Motor Efficiency : Gain  Gain=sm.mu_motor
  Motor Controller : Subsystem  Commented=on
  Motor Electromagnetism : Subsystem  Commented=on
  Rotor Damping : Gain  Gain=sm.b_rotor
  Rotor and Gearing : Subsystem
  Sum : Sum  Inputs=++|
  Sum2 : Sum  Inputs=+|-
  Sum3 : Sum  Inputs=|+-
  Sum4 : Sum  Inputs=+|-
  Sum5 : Sum  Inputs=|++
  Torque Limiter (outside) 2 : Saturate  UpperLimit=sm.LEG_MTR_MAX_TORQUE  LowerLimit=-sm.LEG_MTR_MAX_TORQUE  ZeroCross=off
      settings: AttributesFormatString=Hi: %<UpperLimit>\nLo: %<LowerLimit>
  Rotor Joint Conn : PMIOPort  Port=1  Side=Left
  Shin Joint Torque [Nm] : Outport
  Shin Gear [rad] : Outport  Port=2
  wires:
  Continuous Angle/1 -> Sum/2
  Rotor and Gearing/2(Gearhead Velocity [rad/s]) -> Continuous Angle/2, Sum4/1
  Rotor and Gearing/1(Gearhead Position [rad]) -> Continuous Angle/1
  Sum5/1 -> Shin Joint Torque [Nm]/1, Rotor and Gearing/2(Spring Torque [Nm])
  Torque Limiter (outside) 2/1 -> Inverse Gear Ratio1/1
  Rotor and Gearing/3(Rotor Velocity [rad/s]) -> Rotor Damping/1
  Motor Efficiency/1 -> Rotor and Gearing/1(Rotor Torque [Nm])
  Inverse Gear Ratio1/1 -> Inverse Gear Ratio3/1
  Motor Electromagnetism/1(Current [A]) -> Motor Controller/2(Measured Current [A])
  Motor Controller/1(Voltage [V]) -> Motor Electromagnetism/1(Voltage [V])
  Inverse Gear Ratio2/1 -> Sum3/1
  Inverse Gear Ratio3/1 -> Inverse Gear Ratio2/1
  Rotor Damping/1 -> Sum3/2
  Sum3/1 -> Motor Efficiency/1
  Shin Gear Torque [Nm]/1 -> Motor Direction/1
  Sum/1 -> Shin Gear [rad]/1, Sum2/1
  Initial Gear Angle/1 -> Sum/1
  Demux/2 -> Sum4/2
  Demux/1 -> Sum2/2
  Shin Joint [rad rad/s]/1 -> Demux/1
  Sum4/1 -> Gain1/1
  Gain1/1 -> Sum5/2
  Gain/1 -> Sum5/1  "tau_load"
  Sum2/1 -> Gain/1
  Motor Direction/1 -> Torque Limiter (outside) 2/1
  connections:
  Rotor and Gearing/LConn1 -- Rotor Joint Conn/RConn1

== system atrias_original/ATRIAS_sim/Mechanical System Layer/L Leg/Thigh ==
  CS1 to CS2 : sm_lib/Frames and Transforms/Rigid Transform  TranslationMethod=Cartesian  TranslationStandardOffset=0  TranslationLengthUnit=m  TranslationStandardAxis=+Z  TranslationCartesianOffset=[0 -sm.l_seg 0]  TranslationROffset=0  TranslationROffsetUnits=m  TranslationZOffset=0  TranslationZOffsetUnits=m  TranslationThetaOffset=0  TranslationThetaOffsetUnits=deg  RotationMethod=None  RotationAngleUnits=deg  RotationStandardAxis=+Z  RotationAngle=0  RotationArbitraryAxis=[0 0 1]  FollAlignAxisA=+X  BaseAlignAxisA=+Y  FollAlignAxisB=+Y  BaseAlignAxisB=+Z  RotationSequenceAxes=FollowerAxes  RotationSequence=XYX  RotationSequenceAngles=[0 0 0]  RotationSequenceAnglesUnits=deg  RotationMatrix=[1 0 0; 0 1 0; 0 0 1]
  Frame Data : Subsystem
  Solid : sm_lib/Body Elements/Solid  InertiaType=Custom  Mass=sm.m_thigh  MassUnits=kg  CenterOfMass=sm.com_thigh  CenterOfMassUnits=m  MomentsOfInertia=sm.i_thigh_moments  MomentsOfInertiaUnits=kg*m^2  ProductsOfInertia=sm.i_thigh_products  ProductsOfInertiaUnits=kg*m^2  DensityBased=on  Density=1000  DensityUnits=kg/(m^3)  DoExposeReferenceFrame=on  SerializedFrames=<Frames/>  GraphicType=FromGeometry  MarkerShape=Sphere  MarkerSize=10  MarkerSizeUnits=m  GraphicVisPropType=AdvancedVisualProperties  GraphicDiffuseColor=sm.thigh_color_d  GraphicSpecularColor=[0.5 0.5 0.5 1.0]  GraphicAmbientColor=[sm.thigh_color_d*0.5 1.0]  GraphicEmissiveColor=[0.0 0.0 0.0 1.0]  GraphicShininess=128  GraphicOpacity=1.0  GeometryShape=FromFile  RectangleSize=[1 1]  RectangleSizeUnits=m  BrickDimensions=[1 1 1]  BrickDimensionUnits=m  CylinderRadius=1  CylinderRadiusUnits=m  CylinderLength=1  CylinderLengthUnits=m  SphereRadius=1  SphereRadiusUnits=m  EllipsoidRadii=[1 1 1]  EllipsoidRadiiUnits=m  ExtrusionCrossSection=[1 1; -1 1; -1 -1; 1 -1]  ExtrusionCrossSectionUnits=m  ExtrusionLength=1  ExtrusionLengthUnits=m  PolygonNumSides=3  PolygonOuterRadius=1  PolygonOuterRadiusUnits=m  ExtGeomFileType=STL  ExtGeomFileName=../models/thigh.stl  ExtGeomFileUnits=m  RevolutionCrossSection=[1 1; 1 -1; 2 -1; 2 1]  RevolutionCrossSectionUnits=m  RevolutionExtent=Full  RevolutionAngle=180  RevolutionAngleUnits=deg
  CS1 : PMIOPort  Port=1  Side=Left
  CS2 : PMIOPort  Port=2  Side=Right
  connections:
  CS1/RConn1 -- Frame Data/LConn1 -- Solid/RConn1 -- CS1 to CS2/LConn1
  CS2/RConn1 -- CS1 to CS2/RConn1

== system atrias_original/ATRIAS_sim/Mechanical System Layer/L Leg/Thigh SEA ==
  note: Thigh SEA Mechanics
  Thigh Gear Torque [Nm] : Inport
  Thigh Joint [rad rad/s] : Inport  Port=2
  Continuous Angle : mblibv1/Utilities/Continuous Angle  rad=rad  rads=rad/s
      settings: SourceProductName=Simscape Multibody  SourceProductBaseCode=MS
  Demux : Demux  Outputs=2
  Gain : Gain  Gain=sm.k_leg_spring
  Gain1 : Gain  Gain=sm.b_leg_spring
  Initial Gear Angle : Constant  Value=sm.thigh_initial_l+sm.initial_deflection_l
  Inverse Gear Ratio1 : Gain  Gain=1/sm.N
  Inverse Gear Ratio2 : Gain  Gain=sm.Kt_leg
  Inverse Gear Ratio3 : Gain  Gain=1/sm.Kt_leg
  Motor Direction : Gain  Gain=-1
  Motor Efficiency : Gain  Gain=sm.mu_motor
  Motor Controller : Subsystem  Commented=on
  Motor Electromagnetism : Subsystem  Commented=on
  Rotor Damping : Gain  Gain=sm.b_rotor
  Rotor and Gearing : Subsystem
  Sum : Sum  Inputs=++|
  Sum2 : Sum  Inputs=+|-
  Sum3 : Sum  Inputs=|+-
  Sum4 : Sum  Inputs=+|-
  Sum5 : Sum  Inputs=|++
  Torque Limiter (outside) 2 : Saturate  UpperLimit=sm.LEG_MTR_MAX_TORQUE  LowerLimit=-sm.LEG_MTR_MAX_TORQUE  ZeroCross=off
      settings: AttributesFormatString=Hi: %<UpperLimit>\nLo: %<LowerLimit>
  Rotor Joint Conn : PMIOPort  Port=1  Side=Left
  Thigh Joint Torque [Nm] : Outport
  Thigh Gear [rad] : Outport  Port=2
  wires:
  Torque Limiter (outside) 2/1 -> Inverse Gear Ratio1/1
  Rotor and Gearing/3(Rotor Velocity [rad/s]) -> Rotor Damping/1
  Sum5/1 -> Rotor and Gearing/2(Spring Torque [Nm]), Thigh Joint Torque [Nm]/1
  Rotor and Gearing/2(Gearhead Velocity [rad/s]) -> Continuous Angle/2, Sum4/1
  Motor Efficiency/1 -> Rotor and Gearing/1(Rotor Torque [Nm])
  Inverse Gear Ratio1/1 -> Inverse Gear Ratio3/1
  Thigh Gear Torque [Nm]/1 -> Motor Direction/1
  Motor Electromagnetism/1(Current [A]) -> Motor Controller/2(Measured Current [A])
  Motor Controller/1(Voltage [V]) -> Motor Electromagnetism/1(Voltage [V])
  Rotor and Gearing/1(Gearhead Position [rad]) -> Continuous Angle/1
  Continuous Angle/1 -> Sum/2
  Sum/1 -> Sum2/1, Thigh Gear [rad]/1
  Initial Gear Angle/1 -> Sum/1
  Inverse Gear Ratio2/1 -> Sum3/1
  Inverse Gear Ratio3/1 -> Inverse Gear Ratio2/1
  Demux/2 -> Sum4/2
  Demux/1 -> Sum2/2
  Thigh Joint [rad rad/s]/1 -> Demux/1
  Sum4/1 -> Gain1/1
  Gain1/1 -> Sum5/2
  Gain/1 -> Sum5/1  "tau_load"
  Rotor Damping/1 -> Sum3/2
  Sum3/1 -> Motor Efficiency/1
  Sum2/1 -> Gain/1
  Motor Direction/1 -> Torque Limiter (outside) 2/1
  connections:
  Rotor and Gearing/LConn1 -- Rotor Joint Conn/RConn1

== system atrias_original/ATRIAS_sim/Mechanical System Layer/Left Hip Roll Joint/Mechanical Limits  ==
  vphi : Inport
  phi : Inport  Port=2
  Compare To Constant5 : simulink/Logic and Bit Operations/Compare To Constant  relop=<=  const=sm.phi_max_collision  OutDataTypeStr=boolean  ZeroCross=off
  Compare To Zero1 : simulink/Logic and Bit Operations/Compare To Zero  relop=<=  OutDataTypeStr=boolean  ZeroCross=off
  Compare To Zero2 : simulink/Logic and Bit Operations/Compare To Zero  relop=<=  OutDataTypeStr=boolean  ZeroCross=off
  Constant1 : Constant  Value=sm.phi_roll_min
  Constant2 : Constant  Value=sm.phi_roll_max
  Enabled Subsystem : Subsystem  TreatAsAtomicUnit=on
  Gain2 : Gain  Gain=-1
  Logical Operator : Logic  Operator=OR  Inputs=1  AllPortsSameDT=off  OutDataTypeStr=boolean
  Mux : Mux  Inputs=2
  Roll Max Collision Model : Subsystem
  Roll Min Collision Model : Subsystem
  Stop Simulation6 : Stop
  Sum1 : Sum  Inputs=-+|
  Sum11 : Sum  Inputs=-|+
  Sum5 : Sum  Inputs=+-|
  tau_reaction : Outport
  wires:
  Gain2/1 -> Roll Max Collision Model/2(vphi [rad/s])
  vphi/1 -> Gain2/1, Roll Min Collision Model/2(vphi [rad/s])
  Roll Max Collision Model/1(tau_interaction[Nm]) -> Sum11/1
  Compare To Zero2/1 -> Roll Max Collision Model/Enable
  Sum5/1 -> Roll Max Collision Model/1(phi [rad]), Compare To Zero2/1, [col_hip_max]
  Constant2/1 -> Sum5/1
  Compare To Constant5/1 -> Logical Operator/1, Enabled Subsystem/1(Col_Flags)
  Constant1/1 -> Sum1/1
  Sum11/1 -> tau_reaction/1
  [col_hip_min] -> Mux/2
  Mux/1 -> Compare To Constant5/1
  [col_hip_max] -> Mux/1
  Logical Operator/1 -> Stop Simulation6/1, Enabled Subsystem/Enable
  phi/1 -> Sum5/2, Sum1/2
  Compare To Zero1/1 -> Roll Min Collision Model/Enable
  Roll Min Collision Model/1(tau_interaction[Nm]) -> Sum11/2
  Sum1/1 -> Roll Min Collision Model/1(phi [rad]), Compare To Zero1/1, [col_hip_min]

== system atrias_original/ATRIAS_sim/Mechanical System Layer/R Ground Contact/Angle Range Map1 ==
  "[-pi, pi]" : Inport
  Constant : Constant  Value=2*pi
  Sum3 : Sum  Inputs=|++
  Switch : Switch  ZeroCross=off
  "[0,2*pi]" : Outport
  wires:
  "[-pi, pi]"/1 -> Sum3/1, Switch/1, Switch/2
  Sum3/1 -> Switch/3
  Constant/1 -> Sum3/2
  Switch/1 -> "[0,2*pi]"/1

== system atrias_original/ATRIAS_sim/Mechanical System Layer/R Ground Contact/Ground Friction Model ==
  note: Transverse Ground Friction Model
  note: Normal Ground Stiction Model
  delta normal [m] : Inport
  vnormal [m/s] : Inport  Port=2
  x [m] : Inport  Port=3
  vx [m/s] : Inport  Port=4
  z [m] : Inport  Port=5
  vz [m/s] : Inport  Port=6
  Contact! : EnablePort  StatesWhenEnabling=reset
  Data Type Conversion : DataTypeConversion  OutDataTypeStr=double
  Friction Switch : Subsystem
  Gain3 : Gain  Gain=sm.k_gy
  Gain4 : Gain  Gain=1/sm.v_gy_max
  Logical Operator : Logic  Operator=NOT  AllPortsSameDT=off  OutDataTypeStr=boolean
  Mux1 : Mux  Inputs=2
  Sum1 : Sum
  Sum2 : Sum
  normal-Axis Ground Force : Fcn  Expr="- u(1)  *  (1-u(2)) * (u(2)<1)"
  t-Axis Kinetic Friction Model : Subsystem
  t-Axis Static Friction Model : Subsystem
  FxFriction [N] : Outport  OutputWhenDisabled=reset  InitialOutput=0
      settings: AttributesFormatString=initial = '%<InitialOutput>'\nwhen\ndisabled\n'%<OutputWhenDisabled>'
  FyFriction [N] : Outport  Port=2  OutputWhenDisabled=reset  InitialOutput=0
      settings: AttributesFormatString=initial = '%<InitialOutput>'\nwhen\ndisabled\n'%<OutputWhenDisabled>'
  Fn_Ground[N] : Outport  Port=3  OutputWhenDisabled=reset  InitialOutput=0
      settings: AttributesFormatString=initial = '%<InitialOutput>'\nwhen disabled = '%<OutputWhenDisabled>'
  Stiction! : Outport  Port=4  OutputWhenDisabled=reset  InitialOutput=0
      settings: AttributesFormatString=initial = '%<InitialOutput>'\nwhen\ndisabled\n'%<OutputWhenDisabled>'
  wires:
  normal-Axis Ground Force/1 -> t-Axis Static Friction Model/1(F_Normal [N]), t-Axis Kinetic Friction Model/5(F_Normal [N]), Fn_Ground[N]/1
  delta normal [m]/1 -> Gain3/1
  vnormal [m/s]/1 -> Gain4/1
  x [m]/1 -> t-Axis Kinetic Friction Model/1(pos_x [m]), t-Axis Static Friction Model/2(pos_x [m])
  vx [m/s]/1 -> t-Axis Kinetic Friction Model/2(vel_x [m/s]), t-Axis Static Friction Model/3(vel_x [m/s])
  t-Axis Kinetic Friction Model/1(posFP_x [m]) -> t-Axis Static Friction Model/6(posFP_x [m])
  t-Axis Kinetic Friction Model/4(Fx_Slide [N]) -> Sum1/2
  t-Axis Static Friction Model/2(Fx_Stick [N]) -> Sum1/1
  Sum1/1 -> FxFriction [N]/1
  Friction Switch/1(Stiction) -> Data Type Conversion/1, Logical Operator/1, t-Axis Static Friction Model/Enable
  t-Axis Static Friction Model/3(Sliding!) -> Friction Switch/1(Slide!)
  t-Axis Kinetic Friction Model/3(Stiction!) -> Friction Switch/2(Stick!)
  Logical Operator/1 -> t-Axis Kinetic Friction Model/Enable
  Mux1/1 -> normal-Axis Ground Force/1
  Gain3/1 -> Mux1/1
  Gain4/1 -> Mux1/2
  t-Axis Static Friction Model/1(Fz_Stick [N]) -> Sum2/1
  t-Axis Kinetic Friction Model/5(Fz_Slide [N]) -> Sum2/2
  Sum2/1 -> FyFriction [N]/1
  t-Axis Kinetic Friction Model/2(posFP_z [m]) -> t-Axis Static Friction Model/7(posFP_z [m])
  z [m]/1 -> t-Axis Static Friction Model/4(pos_z [m]), t-Axis Kinetic Friction Model/3(pos_z [m])
  vz [m/s]/1 -> t-Axis Kinetic Friction Model/4(vel_z [m/s]), t-Axis Static Friction Model/5(vel_z [m/s])
  Data Type Conversion/1 -> Stiction!/1

== system atrias_original/ATRIAS_sim/Mechanical System Layer/R Ground Contact/Tranverse Component ==
  "x, y, z" : Inport
  boom yaw [rad] : Inport  Port=2
  Demux1 : Demux  Outputs=3
  Product : Product
  Product1 : Product
  Sum2 : Sum  Inputs=+|+
  Terminator1 : Terminator
  Trigonometric Function1 : Trigonometry  Operator=cos
  Trigonometric Function2 : Trigonometry
  transverse : Outport
  wires:
  Demux1/3 -> Terminator1/1
  "x, y, z"/1 -> Demux1/1
  Product1/1 -> Sum2/2
  Trigonometric Function1/1 -> Product/2
  boom yaw [rad]/1 -> Trigonometric Function2/1, Trigonometric Function1/1
  Product/1 -> Sum2/1
  Sum2/1 -> transverse/1
  Demux1/1 -> Product/1
  Demux1/2 -> Product1/2
  Trigonometric Function2/1 -> Product1/1
